simulink model "muscle_reflex_model"  (R2019b)
settings: Solver=VariableStepAuto  StartTime=0.0  StopTime=6  RelTol=1e-3
values from neighbouring files (symbols this model uses):
  b_m = 2    [reflex_model_variables.m]
  beta = 100    [reflex_model_variables.m]
  k_m = 50    [reflex_model_variables.m]
  m = 0.1    [reflex_model_variables.m]
  omega = 5    [reflex_model_variables.m]
  tau = 1/300    (= 0.00333333333333)    [reflex_model_variables.m]
  time_delay = 0.02    [reflex_model_variables.m]
settings Model: Creator=User  LastModifiedBy=User

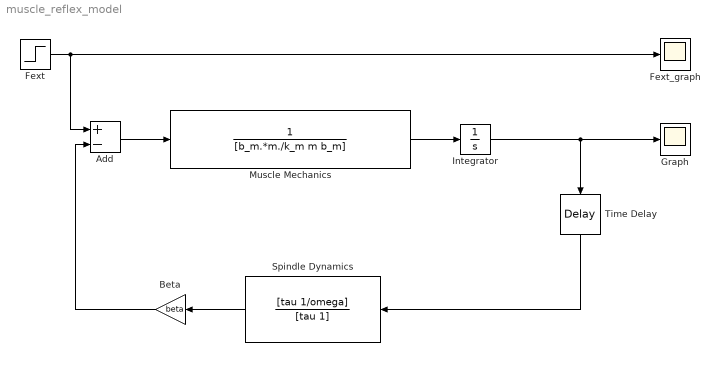
== system muscle_reflex_model ==
  Add : Sum  Inputs=+-
  Beta : Gain  Gain=beta
  Fext : Step  SampleTime=0
  Fext_graph : Scope
  Graph : Scope
  Integrator : Integrator
  Muscle Mechanics : TransferFcn  Numerator=1  Denominator=[b_m.*m./k_m m b_m]
  Spindle Dynamics : TransferFcn  Numerator=[tau 1/omega]  Denominator=[tau 1]
  Time Delay : TransportDelay  DelayTime=time_delay
  wires:
  Muscle Mechanics/1 -> Integrator/1
  Integrator/1 -> Graph/1, Time Delay/1
  Time Delay/1 -> Spindle Dynamics/1
  Spindle Dynamics/1 -> Beta/1
  Beta/1 -> Add/2
  Add/1 -> Muscle Mechanics/1
  Fext/1 -> Fext_graph/1, Add/1
